simulink model "lee_controller"  (R2021b)
settings: Solver=FixedStepAuto  StartTime=0.0  StopTime=inf  FixedStep=dt  RelTol=1e-3  EnableMultiTasking=on
values from neighbouring files (symbols this model uses):
  dt = 1/250    (= 0.004)    [parameters.m]
  ei = [0,0,0]'    [parameters.m]
  eir = [0,0,0]'    [parameters.m]
  g = 9.81    [parameters.m]
  pitch_offset = 0.028    [parameters.m]
  roll_offset = 0.028    [parameters.m]
  thrust_offset = 0.075    [parameters.m]
  yaw_offset = 0.028    [parameters.m]
undefined symbols (not defined in the file or in its folder): AUX, ddz, dev, DiscIntNeverNeededParam, dz, ep, ev, ew, eyaw, f_ext, fz, Main, pwm_output0, pwm_output1, tau, timestamp, z
libraries: px4lib x47, px4uORBlib x14, px4Sensorslib x1
(part 2 of 2)

== matlab function lee_controller/Flight_modes_switch/MATLAB Function ==
  data: flight_mode input; stab_flag output; pos_flag output
function [stab_flag, pos_flag] = block_switch(flight_mode)
    
    stab_flag = boolean(0);
    pos_flag = boolean(0);

    if(flight_mode == 8) %Stabilized
        stab_flag = boolean(1);
        pos_flag = boolean(0);
    elseif (flight_mode == 2) %Position
            pos_flag = boolean(1);
            stab_flag = boolean(0);
    end   
    
end

== matlab function lee_controller/mode sw ==
  data: pos_flag input; rpm output; pos_rpm input; stab_flag input; stab_rpm input
function rpm = fcn(pos_flag, pos_rpm, stab_flag, stab_rpm)

    if pos_flag == boolean(1)
        rpm = pos_rpm;
    elseif stab_flag == boolean(1)
        rpm = stab_rpm;
    else
        rpm = 0.*ones(4,1);
    end

end

== matlab function lee_controller/Drone_pwm_converter/MATLAB Function4 ==
  data: rpm input; pwm output
function pwm = fcn(rpm)

    rpm_max = 8800;
    pwm_max = 2000;
%     pwm_min = 1000;

    pwm = uint16( 1000 + ( (rpm*pwm_max/rpm_max )*100) );

end

== matlab function lee_controller/uORB_reads/MATLAB Function ==
  data: kill_sw input; arm output; arm_cmd input
function arm = check_kill(kill_sw, arm_cmd)

    if(kill_sw)
        arm = boolean(0);
    else
        if(arm_cmd)
            arm = boolean(1);
        else
            arm = boolean(0);
        end
    end


end

== matlab function lee_controller/Enabled Subsystem1/rpm allocation ==
  data: f input; rpm output; M input; A_inv parameter; inv_A input
function rpm = allocation(f, M, A_inv, inv_A)
    rpm = zeros(4,1);
    radsec = zeros(4,1);
    ft = zeros(4,1);
    ft(1) = -f;
    ft(2:4) = M;

%     radsec_squared = A_inv *ft; %from parameters.m
    radsec_squared = inv_A *ft; %from simulink


    %ordine angoli marice m1, m4, m2, m3

    if( f <= 0.05)
        rpm = zeros(4,1);
    else
        for i=1:4
            if(radsec_squared(i) > 0.0)
                radsec(i) = sqrt( radsec_squared(i) );
            else
                radsec(i) = 0.0;
            end
        end

        rpm = radsec.*9.54;
    end


end

== matlab function lee_controller/Enabled Subsystem1/att control ==
  data: eul_des input; omega_des output; q input; Kp_x input; Kp_y input; Kp_z input; yaw_drone output
function [omega_des, yaw_drone] = att_contr(eul_des, q, Kp_x, Kp_y, Kp_z)

    omega_des = zeros(3,1);

    %Mavros uses [x y z w], i use [w x y z]
%     qB = [q(4), q(3), q(2), q(1)]';

    q_drone = q;
    Kp_orien = diag([Kp_x, Kp_y, Kp_z]);

    R_drone = quat2rotm(q_drone);
    yaw_drone = atan2(R_drone(2,1), R_drone(1,1));
    Rz_drone = [cos(yaw_drone), -sin(yaw_drone), 0;
                sin(yaw_drone), cos(yaw_drone), 0;
                0, 0, 1];
    
    qB = rotm2quat( Rz_drone' * R_drone )';

    %quaternion error
    q_des = eul2quat(eul_des', 'XYZ')';
    
    eq = zeros(4,1);
    vB = qB(2:4);
    v_des = q_des(2:4);
    
    n_des = q_des(1);
    nB =qB(1);
    
    eq(1) = n_des * nB + v_des' * vB;
    eq(2:4) = nB*v_des - n_des*vB + cross(v_des, -vB);


    omega_des = Kp_orien * sign(eq(1)) * eq(2:4);
    
end

== matlab function lee_controller/Enabled Subsystem1/rate control ==
  data: omega input; omega_des input; J_xx input; J_yy input; J_zz input; Kd_x input; M_des output; Kd_y input; Kd_z input
function M_des = rate_contr(omega, omega_des, J_xx, J_yy, J_zz, Kd_x, Kd_y, Kd_z)
    M_des = zeros(3,1);
    J = diag([J_xx, J_yy, J_zz]);
    
    Kd_orien = diag([Kd_x, Kd_y, Kd_z]);
    M_des = Kd_orien * (omega_des - omega) + cross(omega, J*omega);

end

== matlab function lee_controller/Setpoints/kill sw ==
  data: cmd input; kill_sw output
function kill_sw = fcn(cmd)

    if(cmd > 1800)
        kill_sw = boolean(1);
    else
        kill_sw = boolean(0);
    end

end

== matlab function lee_controller/Feedback/MATLAB Function ==
  data: q input; eul output; R_mes output
function [eul, R_mes] = or_fb(q)
    
    eul = zeros(1,3);
    R = quat2rotm(q);
    eul(1) = atan2(    R(3,2), R(3,3) );
    eul(2) = atan2( -R(3,1), sqrt( R(3,2)*R(3,2) + R(3,3)*R(3,3)));
    eul(3) = atan2(R(2,1),R(1,1));
    R_mes = R;

end

== matlab function lee_controller/Enabled Subsystem1/inv alloc_matrix ==
  data: kf input; inv_A output; km input; l_arm input
function inv_A  = fcn(kf,km,l_arm)

    inv_A = [-1/(4*kf), -2^(1/2)/(4*l_arm*kf),  2^(1/2)/(4*l_arm*kf),  1/(4*km);
             -1/(4*kf),  2^(1/2)/(4*l_arm*kf), -2^(1/2)/(4*l_arm*kf),  1/(4*km);
             -1/(4*kf),  2^(1/2)/(4*l_arm*kf),  2^(1/2)/(4*l_arm*kf), -1/(4*km);
             -1/(4*kf), -2^(1/2)/(4*l_arm*kf), -2^(1/2)/(4*l_arm*kf), -1/(4*km)];
end

== matlab function lee_controller/Drone_pwm_converter/MATLAB Function1 ==
  settings: updateMethod=DISCRETE  sampleTime=dt
  data: ch6 input; servo_pwm output uint16 size=1
function servo_pwm = fcn(ch6)
    servo_cmd=uint16(0);
    if ch6>=1620
        servo_cmd=1;
    elseif (ch6<1620 && ch6>1420)
        servo_cmd=0;
    else
        servo_cmd=-1;
    end

    servo_pwm=uint16(1520+servo_cmd*50);
  
end

== matlab function lee_controller/Subsystem1/Bit sign ==
  settings: sampleTime=dt
  data: u input; y output size=1
function y = fcn(u)
  
  x=dec2bin(u,8);
  
  y=bin2dec(x);
end

== matlab function lee_controller/LEE_CONTROLLER/lee pos ==
  data: x_drone input; f output; ex output; ev output; b3d output; v_drone input; x_des input; v_des input; a_des input; R_drone input; g parameter; kp_x input; kp_y input; kp_z input; kd_x input; kd_y input; kd_z input; ki_x input; ki_y input; ki_z input; c1 input; mass input; dt parameter; sat input; ei parameter; sat_flag output
function [f, ex, ev, b3d, sat_flag] = position_control(x_drone, v_drone, x_des, v_des, a_des, R_drone, g, kp_x, kp_y, kp_z, kd_x, kd_y, kd_z, ki_x, ki_y, ki_z, c1, mass, dt, sat, ei)
    sat_flag = boolean(false);
    
    Kp_mat = [kp_x,0,0;
             0,kp_y,0;
              0,0,kp_z];

    Kd_mat = [kd_x,0,0;
             0,kd_y,0;
              0,0,kd_z];

    Ki_mat = [ki_x,0,0;
              0,ki_y,0;
               0,0,ki_z];


    ex = x_drone - x_des;
    ev = v_drone - v_des;
    e3 = [0;0;1];
   
    ei = ei + dt*(ev+c1*ex);
    for i=1:3
      if (ei(i)>sat)
        ei(i) = sat; 
        sat_flag = boolean(true);
      end
      if(ei(i)<-sat)
        ei(i)=-sat; 
        sat_flag = boolean(true);
      end
      if(ei(i)>=-sat && ei(i)<=sat )
        sat_flag = boolean(false);
      end
    end
    
    PD =  -Kp_mat*ex - Kd_mat*ev -Ki_mat*ei - mass*g*e3 + mass*a_des ;

    b3d = double(-PD/norm(PD));
    f = double(dot(-PD, R_drone*e3));

end

== matlab function lee_controller/LEE_CONTROLLER/rpm_pos allocation ==
  data: f input; rpm output; M input; A_inv parameter; inv_A input
function rpm = allocation(f, M, A_inv, inv_A)
    rpm = zeros(4,1);
    radsec = zeros(4,1);
    ft = zeros(4,1);
    ft(1) = -f;
    ft(2:4) = M;

%     radsec_squared = A_inv *ft; %from parameters.m
    radsec_squared = inv_A *ft; %from simulink


    %ordine angoli marice m1, m4, m2, m3

    if( f <= 0.05)
        rpm = zeros(4,1);
    else
        for i=1:4
            if(radsec_squared(i) > 0.0)
                radsec(i) = sqrt( radsec_squared(i) );
            else
                radsec(i) = 0.0;
            end
        end

        rpm = radsec.*9.54;
    end


end

== matlab function lee_controller/LEE_CONTROLLER/lee att ==
  data: b3d input; M output; des_yaw input; R_mes input; omega input; omega_d input; omega_d_dot input; eR output; kp_roll input; kp_pitch input; kp_yaw input; kd_roll input; kd_pitch input; kd_yaw input; ki_roll input; ki_pitch input; ki_yaw input; c2 input; J_xx input; J_yy input; J_zz input; dt parameter; eir parameter; e_omega output
function [M, eR, e_omega] = attitude_control(b3d, des_yaw, R_mes, omega, omega_d, omega_d_dot, kp_roll, kp_pitch, kp_yaw, kd_roll, kd_pitch, kd_yaw, ki_roll, ki_pitch, ki_yaw, c2, J_xx, J_yy, J_zz, dt, eir)
    
    M = double(zeros(3,1)); 
    J = double(zeros(3,3));
    
    J = [J_xx,0,0;
         0,J_yy,0;
         0,0,J_zz];

    Kr = [kp_roll,0,0;
         0,kp_pitch,0;
          0,0,kp_yaw];

    Komega = [kd_roll,0,0;
             0,kd_pitch,0;
              0,0,kd_yaw];

    Komegai = [ki_roll,0,0;
              0,ki_pitch,0;
               0,0,ki_yaw];
    
    omega_hat = [0, -omega(3), omega(2);
                 omega(3), 0, -omega(1);
                -omega(2), omega(1), 0];

    
    b1d = [cos(des_yaw); sin(des_yaw); 0];
    b2d_cross = cross(b3d, b1d);
    b2d = b2d_cross/norm(b2d_cross);

    Rd = [cross(b2d,b3d), b2d, b3d];

    R_err = 0.5 * ( Rd'*R_mes - R_mes'*Rd );

    eR = [R_err(3,2); R_err(1,3); R_err(2,1)];

    e_omega = omega - R_mes'*Rd*omega_d;

    eir = eir +dt*(e_omega+c2*eR);

    M = double(-Kr*eR -Komega*e_omega -Komegai*eir + cross(omega, J*omega) -J* ( omega_hat*R_mes'*Rd*omega_d - R_mes'*Rd*omega_d_dot ));    

end
